simulink model "EthanModel"  (R2019b)
settings: Solver=VariableStepAuto  StartTime=0.0  StopTime=10  RelTol=1e-3
values from neighbouring files (symbols this model uses):
  A = double(round(subs(J_x,   [states, inputs], [trim_state, trim_input])*1000)/1000)    [matlab_init.m]
  A_double = [0 1; 0 0]    [matlab_init.m]
  A_s_double = eval(subs(Ad_double,Ts))    [matlab_init.m]
  A_s_single = eval(subs(Ad_single,Ts))    [matlab_init.m]
  A_single = [0]    [matlab_init.m]
  Aaileron = A(5:8,5:8)    [matlab_init.m]
  Aelevator = A(1:4,1:4)    [matlab_init.m]
  Arudder = A(11:12,11:12)    [matlab_init.m]
  Athrust = A(9:10,9:10)    [matlab_init.m]
  B = B*MotorMix    [matlab_init.m]
  B_double = [0; 1]    [matlab_init.m]
  B_s_double = eval(subs(Bd_double,Ts))    [matlab_init.m]
  B_s_single = eval(subs(Bd_single,Ts))    [matlab_init.m]
  B_single = [1]    [matlab_init.m]
  Baileron = B(5:8,3)    [matlab_init.m]
  Belevator = B(1:4,2)    [matlab_init.m]
  Brudder = B(11:12,4)    [matlab_init.m]
  Bthrust = B(9:10,1)    [matlab_init.m]
  C = double(round(subs(J_y,   [states, inputs], [trim_state, trim_input])*1000)/1000)    [matlab_init.m]
  C_double = [1 0]    [matlab_init.m]
  C_P = 0.041    [matlab_init.m]
  C_rollpitch = rho*prop_dia^4*prop_dist/sqrt(2)*[                 1  -1  -1   1 ;                 1   1  -1  -1 ;                 0   0   0   0 ; ]    [matlab_init.m]
  C_single = [1]    [matlab_init.m]
  C_T = [0.069075;4.95e-05]    [matlab_init.m]
  C_yaw = rho*prop_dia^5/(2*pi)*[                 0   0   0   0 ;                 0   0   0   0 ;                -1   1  -1   1 ; ]    [matlab_init.m]
  Caileron = [0 1 0 0; 0 0 0 1]    [matlab_init.m]
  Celevator = [0 1 0 0; 0 0 0 1]    [matlab_init.m]
  Crudder = [0 1]    [matlab_init.m]
  Cthrust = [ 1 0; 0 0]    [matlab_init.m]
  D = D*MotorMix    [matlab_init.m]
  D_double = [0]    [matlab_init.m]
  D_single = [0]    [matlab_init.m]
  Daileron = [0 ; 0]    [matlab_init.m]
  Delevator = [0 ; 0]    [matlab_init.m]
  Drudder = 0    [matlab_init.m]
  Dthrust = [0 ; D(4,1)]    [matlab_init.m]
  g = [0;0;UAV_mass*9.81]    [matlab_init.m]
  I_flip = eye(12)    [matlab_init.m]
  J = [      Jxx   0   0 ;       0   Jyy  0 ;       0    0  Jzz; ]    [matlab_init.m]
  Jinv = inv(J)    [matlab_init.m]
  L_double = lqe(A_double, G_double, C_double, q_double, r_double, 0)    [matlab_init.m]
  L_single = lqe(A_single, G_single, C_single, q_single, r_single, 0)    [matlab_init.m]
  measurement_noise = 0.1    [matlab_init.m]
  MotorMix = [                 1  1  1 -1 ;                 1  1 -1  1 ;                 1 -1 -1 -1 ;                 1 -1  1  1 ; ]    [matlab_init.m]
  omega_c = 2*pi *20    (= 125.663706144)    [matlab_init.m]
  process_noise = 0.05    [matlab_init.m]
  Prop_H = 2*pi*Jprop*[               0  0  0  0 ;               0  0  0  0 ;               1 -1  1 -1 ; ]    [matlab_init.m]
  q_single = cov(out.In_Out_Data{1}.Values.Data)*10000000000000    [matlab_init.m]
  r_single = cov(out.In_Out_Data{2}.Values.Data)    [matlab_init.m]
  tau2 = 1/(20*pi)    (= 0.0159154943092)    [matlab_init.m]
  Thrust_Sum = rho*prop_dia^4*[                 0   0   0   0 ;                 0   0   0   0 ;                -1  -1  -1  -1 ; ]    [matlab_init.m]
  trim_input = [293,293,293,293]    [matlab_init.m]
  trim_state = [0,0,0,0,0,0,0,0,0,0,0,0]    [matlab_init.m]
  Ts = 0.005    [matlab_init.m]
  UAV_mass = 0.068    [matlab_init.m]
undefined symbols (not defined in the file or in its folder): DiscIntNeverNeededParam, Discrete, Time
libraries: ctrlSharedLib x10, simulink x4, vrlib x3, dspmtrx3 x1
(part 2 of 2)

== system EthanModel/Nonlinear System Dynamics/Calculate Velocity/Calculate_Thrust ==
  note: $F_{T} = \sum_{i=1}^4[0;0;C_{T}.*n.^2]$
  n : Inport
  Constant15 : Constant  Value=C_T(1)
  Constant16 : Constant  Value=2
  Gain4 : Gain  Gain=Thrust_Sum  Multiplication=Matrix(K*u)
      settings: AttributesFormatString=%<Gain>
  Gain5 : Gain  Gain=C_T(2)
  Power : Math  Operator=pow  SignedPower=off  SaturateOnIntegerOverflow=on
  Product2 : Product
  Sum1 : Sum  Inputs=++|
  F_T : Outport
  wires:
  Constant15/1 -> Sum1/1
  Gain4/1 -> F_T/1  "F_T"
  n/1 -> Power/1, Gain5/1
  Power/1 -> Product2/2  "props squared"
  Gain5/1 -> Sum1/2
  Sum1/1 -> Product2/1
  Product2/1 -> Gain4/1
  Constant16/1 -> Power/2

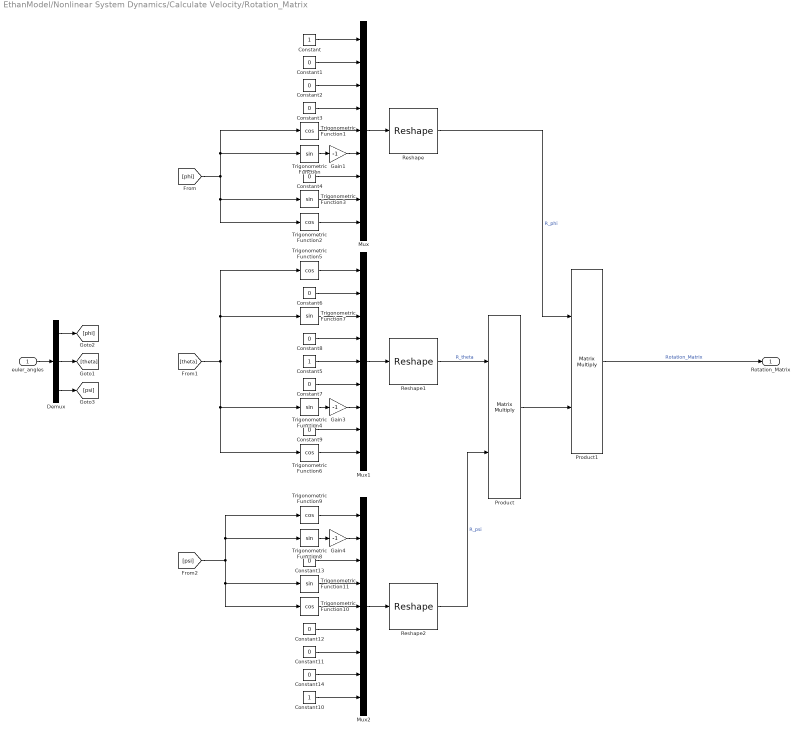
== system EthanModel/Nonlinear System Dynamics/Calculate Velocity/Rotation_Matrix ==
  "euler_angles " : Inport
  Constant : Constant
  Constant{1..4,6..9,11..14} (12 alike) : Constant  Value=0
  Constant10 : Constant
  Constant5 : Constant
  Demux : Demux  Outputs=3
  Gain1 : Gain  Gain=-1
  Gain3 : Gain  Gain=-1
  Gain4 : Gain  Gain=-1
  Mux : Mux  Inputs=9
  Mux1 : Mux  Inputs=9
  Mux2 : Mux  Inputs=9
  Product : Product  Multiplication=Matrix(*)
  Product1 : Product  Multiplication=Matrix(*)
  Reshape : Reshape  OutputDimensionality=Customize  OutputDimensions=[3,3]
  Reshape1 : Reshape  OutputDimensionality=Customize  OutputDimensions=[3,3]
  Reshape2 : Reshape  OutputDimensionality=Customize  OutputDimensions=[3,3]
  Trigonometric Function{,3..4,7..8,11} (6 alike) : Trigonometry
  Trigonometric Function{1..2,5..6,9..10} (6 alike) : Trigonometry  Operator=cos
  Rotation_Matrix : Outport
  wires:
  Constant9/1 -> Mux1/8
  Constant11/1 -> Mux2/7
  Trigonometric Function1/1 -> Mux/5
  Trigonometric Function3/1 -> Mux/8
  Constant5/1 -> Mux1/5
  Trigonometric Function7/1 -> Mux1/3
  Reshape/1 -> Product1/1  "R_phi"
  Mux1/1 -> Reshape1/1
  Trigonometric Function8/1 -> Gain4/1
  Constant7/1 -> Mux1/6
  Trigonometric Function2/1 -> Mux/9
  [phi] -> Trigonometric Function2/1, Trigonometric Function3/1, Trigonometric Function1/1, Trigonometric Function/1
  Trigonometric Function6/1 -> Mux1/9
  Constant12/1 -> Mux2/6
  Trigonometric Function4/1 -> Gain3/1
  [theta] -> Trigonometric Function7/1, Trigonometric Function5/1, Trigonometric Function4/1, Trigonometric Function6/1
  Reshape2/1 -> Product/2  "R_psi"
  Trigonometric Function/1 -> Gain1/1
  Product/1 -> Product1/2
  Trigonometric Function5/1 -> Mux1/1
  Trigonometric Function9/1 -> Mux2/1
  Mux/1 -> Reshape/1
  Constant/1 -> Mux/1
  Constant3/1 -> Mux/4
  Constant6/1 -> Mux1/2
  Mux2/1 -> Reshape2/1
  Constant2/1 -> Mux/3
  Constant1/1 -> Mux/2
  [psi] -> Trigonometric Function11/1, Trigonometric Function10/1, Trigonometric Function9/1, Trigonometric Function8/1
  Constant8/1 -> Mux1/4
  Constant4/1 -> Mux/7
  Constant13/1 -> Mux2/3
  Trigonometric Function11/1 -> Mux2/4
  Constant10/1 -> Mux2/9
  Reshape1/1 -> Product/1  "R_theta"
  Constant14/1 -> Mux2/8
  Trigonometric Function10/1 -> Mux2/5
  Product1/1 -> Rotation_Matrix/1  "Rotation_Matrix"
  Demux/3 -> [psi]
  Demux/2 -> [theta]
  "euler_angles "/1 -> Demux/1
  Demux/1 -> [phi]
  Gain3/1 -> Mux1/7
  Gain1/1 -> Mux/6
  Gain4/1 -> Mux2/2

== matlab function EthanModel/Drone Visualization ==
  data: T input
function drone_visualization(T)

%% /// IMPORTANT ///
%T is array that hold states
%ZED is pointing downwards
%MAKE A MATLAB FUNCTION BLOCK IN SIMULINK
%PASS IN THE NED STATES AND EULER ANGLES
%ADJUST THE STATES AS NECESSARY
%the drone is .18 meters by .18 meters

%the simulation will run MUCH slower while running the visualization
%you can comment out the function block to run the simulation quicker

%% constants
d = .18/2;
c1 = [d; d; 0]; %motor coordinates compared to center of drone
c2 = [d; -d; 0];
c3 = -c1;
c4 = -c2;

    %% adjust indices to get [X; Y; Z] and phi, theta, psi
    XYZ =  [T(1); ...
            T(2); ...
           -T(3)];
    phi =   T(7);
    theta = T(8);
    psi =   T(9);
    %%Defining rotation matrices
    Rx = [1 0 0; 0 cos(theta) sin(theta); 0 -sin(theta) cos(theta)];
    Ry = [cos(phi) 0 -sin(phi); 0 1 0; sin(phi) 0 cos(phi)];
    Rz = [cos(psi) sin(psi) 0; -sin(psi) cos(psi) 0; 0 0 1];
    b1 = Rz*Ry*Rx*c1;
    b2 = Rz*Ry*Rx*c2;
    b3 = Rz*Ry*Rx*c3;
    b4 = Rz*Ry*Rx*c4;
    m1 = XYZ + b1;
    m2 = XYZ + b2;
    m3 = XYZ + b3;
    m4 = XYZ + b4;
    P1 = [m1 m3];
    P2 = [m2 m4];
    P3 = [m1 m2];
    P4 = [m3 m4];

    %%displaying the drone
    plot3(P1(1,:),P1(2,:),P1(3,:),'k-', 'linewidth', 2);
    axis([-3 3 -3 3 -0 3]);
    xlabel('X Axis [Meters]')
    ylabel('Y Axis [Meters]')
    zlabel('Height [Meters]')
    hold on;
    grid on;
    plot3(P2(1,:),P2(2,:),P2(3,:),'k-', 'linewidth', 2);
    plot3(P3(1,:),P3(2,:),P3(3,:),'ob', 'linewidth', 1);
    plot3(P4(1,:),P4(2,:),P4(3,:),'ok', 'linewidth', 1);
    hold off
end
